simulink model "untitled"  (Simulink 9.2)
settings: Solver=ode45  StartTime=0.0  StopTime=1000  FixedStep=100000  RelTol=1e-3  EnableMultiTasking=on
settings Model: Creator=student  LastModifiedBy=murad
settings OptimizationCC: ExpressionDepthLimit=2147483647
settings DebuggingCC: SolverPrmCheckMsg=warning

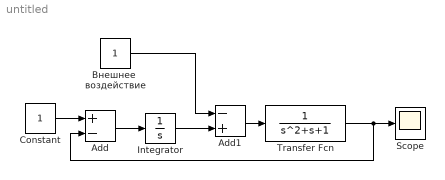
== system untitled ==
  Add : Sum  Inputs=+-
  Add1 : Sum  Inputs=-+
  Constant : Constant
  Integrator : Integrator
  Scope : Scope
  Transfer Fcn : TransferFcn  Denominator=[1 1 1]
  Внешнее  воздействие : Constant
  wires:
  Constant/1 -> Add/1
  Add/1 -> Integrator/1
  Transfer Fcn/1 -> Add/2, Scope/1
  Integrator/1 -> Add1/2
  Внешнее  воздействие/1 -> Add1/1
  Add1/1 -> Transfer Fcn/1
